simulink model "setPoint_sim"  (R2024a)
settings: Solver=VariableStepAuto  StartTime=0.0  StopTime=t_sim  RelTol=1e-3
undefined symbols (not defined in the file): a, g, h_des, K
settings Model: Creator=lorenzo  LastModifiedBy=lorenzo

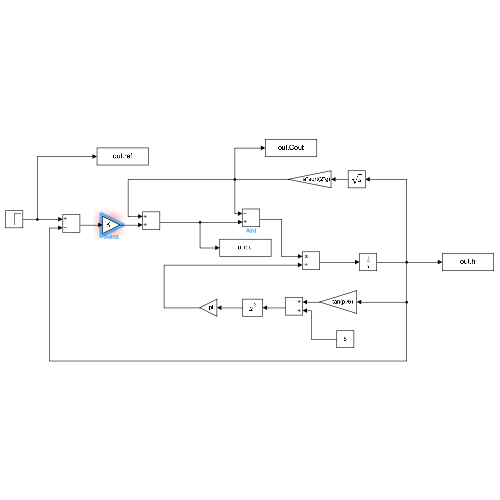
[thumbnail: Simulink's stored preview of the top-level diagram]
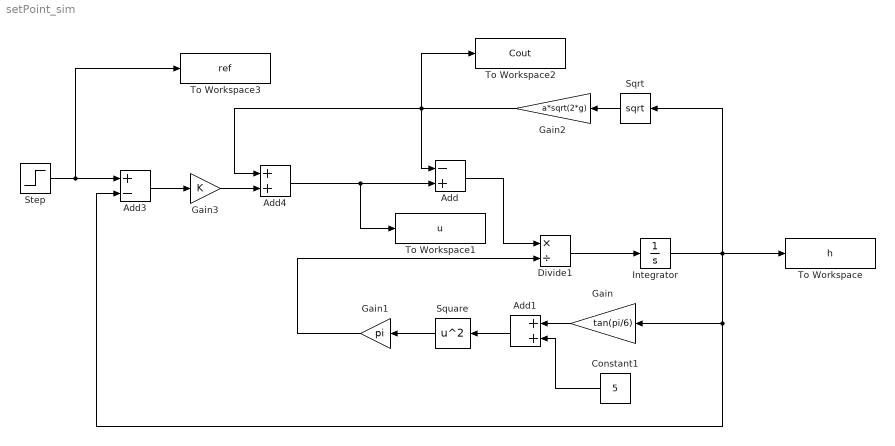
== system setPoint_sim ==
  Add : Sum  Inputs=-+
  Add1 : Sum
  Add3 : Sum  Inputs=+-
  Add4 : Sum
  Constant1 : Constant  Value=5
  Divide1 : Product  Inputs=*/
  Gain : Gain  Gain=tan(pi/6)
  Gain1 : Gain  Gain=pi
  Gain2 : Gain  Gain=a*sqrt(2*g)
  Gain3 : Gain  Gain=K
  Integrator : Integrator
  Sqrt : Sqrt
  Square : Math  Operator=square
  Step : Step  Time=0  After=h_des  SampleTime=0
  To Workspace : ToWorkspace  VariableName=h  SaveFormat=Timeseries  SampleTime=-1
  To Workspace1 : ToWorkspace  VariableName=u  SaveFormat=Timeseries  SampleTime=-1
  To Workspace2 : ToWorkspace  VariableName=Cout  SaveFormat=Timeseries  SampleTime=-1
  To Workspace3 : ToWorkspace  VariableName=ref  SaveFormat=Timeseries  SampleTime=-1
  wires:
  Integrator/1 -> Sqrt/1, To Workspace/1, Gain/1, Add3/2
  Square/1 -> Gain1/1
  Gain/1 -> Add1/1
  Add1/1 -> Square/1
  Constant1/1 -> Add1/2
  Sqrt/1 -> Gain2/1
  Gain2/1 -> Add4/1, To Workspace2/1, Add/1
  Gain1/1 -> Divide1/2
  Divide1/1 -> Integrator/1
  Add/1 -> Divide1/1
  Step/1 -> To Workspace3/1, Add3/1
  Add3/1 -> Gain3/1
  Add4/1 -> Add/2, To Workspace1/1
  Gain3/1 -> Add4/2
